simulink model "sl_braitenberg_1d"  (R2020b)
settings: Solver=VariableStepAuto  StartTime=0.0  StopTime=200  RelTol=1e-3  EnableMultiTasking=on
undefined symbols (not defined in the file or in its folder): SE2
libraries: roblocks x1, simulink x1
settings Model: Creator=corkep  LastModifiedBy=cr-ja
settings DataIOCC: LimitDataPoints=on  SaveFormat=Array  SaveOutput=off  SaveState=on  ReturnWorkspaceOutputs=off
settings OptimizationCC: LifeSpan=inf
settings DebuggingCC: AllowSymbolicDim=off  SFUnexpectedBacktrackingDiag=warning  SFNoUnconditionalDefaultTransitionDiag=warning  SFExecutionAtInitializationDiag=none  ArithmeticOperatorsInVariantConditions=warning
settings HardwareCC: ProdWordSize=32
settings ModelReferenceCC: PropagateSignalLabelsOutOfModel=off
settings SFSimCC: SimUseLocalCustomCode=off  CustomCodeUndefinedFunction=UseInterfaceOnly
settings RTWCC: RTWUseLocalCustomCode=off
settings CodeAppCC: StateflowObjectComments=on
settings GRTTargetCC: TargetLangStandard=C89/C90 (ANSI)
settings ConfigComp: CovMetricSettings=dw  CovSaveCumulativeToWorkspaceVar=on  CovSaveSingleToWorkspaceVar=on  CovExternalEMLEnable=off

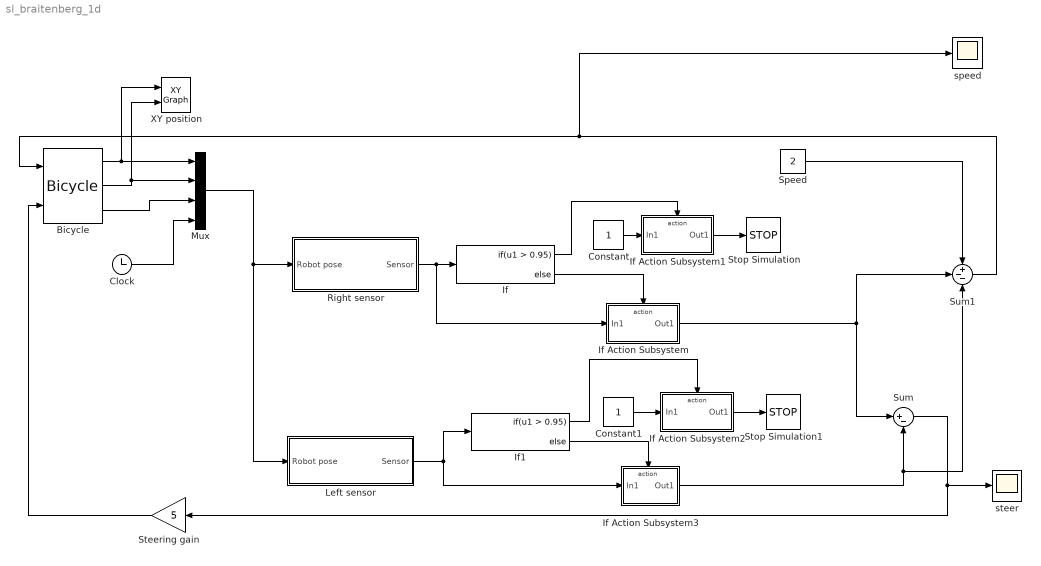
== system sl_braitenberg_1d ==
  Bicycle : roblocks/Vehicles/Bicycle  vlim=1  accel=1  alim=2  steer_rate=Inf  L=1  x0=[0, 0, 0]
  Clock : Clock
  Constant : Constant
  Constant1 : Constant
  If : If  IfExpression=u1 > 0.95
  If Action Subsystem : Subsystem  TreatAsAtomicUnit=on
  If Action Subsystem1 : Subsystem  TreatAsAtomicUnit=on
  If Action Subsystem2 : Subsystem  TreatAsAtomicUnit=on
  If Action Subsystem3 : Subsystem  TreatAsAtomicUnit=on
  If1 : If  IfExpression=u1 > 0.95
  Left sensor : Subsystem  mask{dx=0, dy=-2, sensorfunc=@sensorfield_1d}
      mask prompts: dx "Sensor position x"; dy "Sensor position y"; sensorfunc "Sensor function"
  Mux : Mux
  Right sensor : Subsystem  mask{dx=0, dy=2, sensorfunc=@sensorfield_1d}
      mask prompts: dx "Sensor position x"; dy "Sensor position y"; sensorfunc "Sensor function"
  Speed : Constant  Value=2
  Steering gain : Gain  Gain=5
  Stop Simulation : Stop
  Stop Simulation1 : Stop
  Sum : Sum  Inputs=|+-
  Sum1 : Sum  Inputs=+--
  XY position : simulink/Sinks/XY Graph  xmin=0  xmax=100  ymin=0  ymax=100  st=-1
  speed : Scope
  steer : Scope
  wires:
  Bicycle/1 -> XY position/1, Mux/1
  Bicycle/2 -> XY position/2, Mux/2
  Bicycle/3 -> Mux/3
  Mux/1 -> Left sensor/1(Robot pose), Right sensor/1(Robot pose)
  Sum/1 -> steer/1, Steering gain/1
  If Action Subsystem3/1(Out1) -> Sum/2, Sum1/3
  Sum1/1 -> Bicycle/1, speed/1
  Speed/1 -> Sum1/1
  Steering gain/1 -> Bicycle/2
  Clock/1 -> Mux/4
  If/1 -> If Action Subsystem1/Action
  If1/1 -> If Action Subsystem2/Action
  If Action Subsystem/1(Out1) -> Sum/1, Sum1/2
  If/2 -> If Action Subsystem/Action
  If Action Subsystem1/1(Out1) -> Stop Simulation/1
  Right sensor/1(Sensor) -> If Action Subsystem/1(In1), If/1
  If1/2 -> If Action Subsystem3/Action
  If Action Subsystem2/1(Out1) -> Stop Simulation1/1
  Left sensor/1(Sensor) -> If Action Subsystem3/1(In1), If1/1
  Constant/1 -> If Action Subsystem1/1(In1)
  Constant1/1 -> If Action Subsystem2/1(In1)

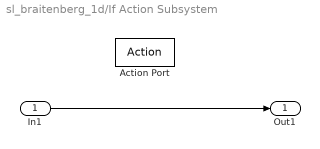
== system sl_braitenberg_1d/If Action Subsystem ==
  In1 : Inport
  Action Port : ActionPort  ActionPortLabel=else
  Out1 : Outport
  wires:
  In1/1 -> Out1/1

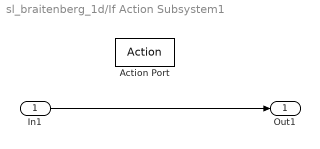
== system sl_braitenberg_1d/If Action Subsystem1 ==
  In1 : Inport
  Action Port : ActionPort  ActionPortLabel=if(u1 > 0.95)
  Out1 : Outport
  wires:
  In1/1 -> Out1/1

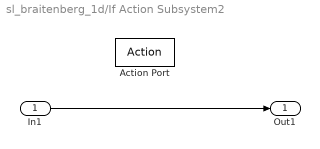
== system sl_braitenberg_1d/If Action Subsystem2 ==
  In1 : Inport
  Action Port : ActionPort  ActionPortLabel=if(u1 > 0.95)
  Out1 : Outport
  wires:
  In1/1 -> Out1/1

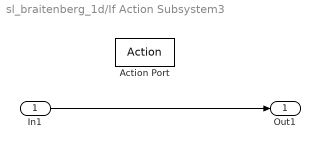
== system sl_braitenberg_1d/If Action Subsystem3 ==
  In1 : Inport
  Action Port : ActionPort  ActionPortLabel=else
  Out1 : Outport
  wires:
  In1/1 -> Out1/1

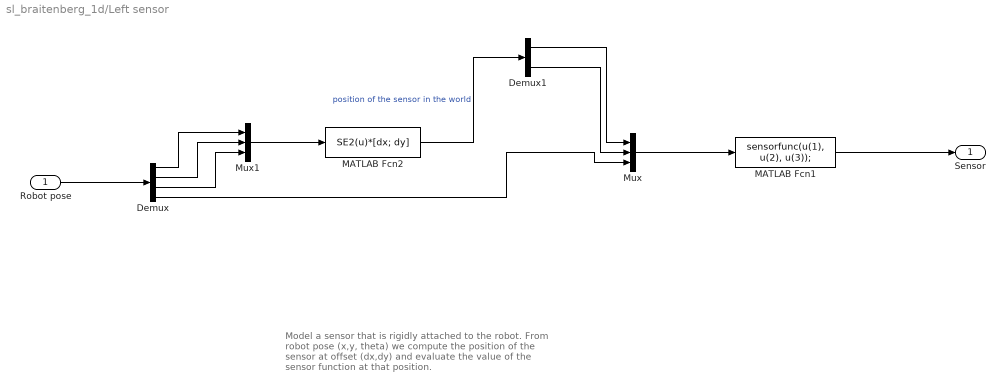
== system sl_braitenberg_1d/Left sensor ==
  note: Model a sensor that is rigidly attached to the robot.
      | From robot pose (x,y, theta) we compute the position of
      | the sensor at offset (dx,dy) and evaluate the value
      | of the sensor function at that position.
  Robot pose : Inport
  Demux : Demux
  Demux1 : Demux  Outputs=2
  MATLAB Fcn1 : MATLABFcn  MATLABFcn=sensorfunc(u(1), u(2), u(3));  OutputDimensions=1
  MATLAB Fcn2 : MATLABFcn  MATLABFcn=SE2(u)*[dx; dy]
  Mux : Mux  Inputs=3
  Mux1 : Mux  Inputs=3
  Sensor : Outport
  wires:
  MATLAB Fcn1/1 -> Sensor/1
  Demux/3 -> Mux1/3
  Demux1/1 -> Mux/1
  Demux/2 -> Mux1/2
  Demux/4 -> Mux/3
  Demux/1 -> Mux1/1
  Mux1/1 -> MATLAB Fcn2/1
  MATLAB Fcn2/1 -> Demux1/1  "position of the sensor in the world"
  Robot pose/1 -> Demux/1
  Mux/1 -> MATLAB Fcn1/1
  Demux1/2 -> Mux/2

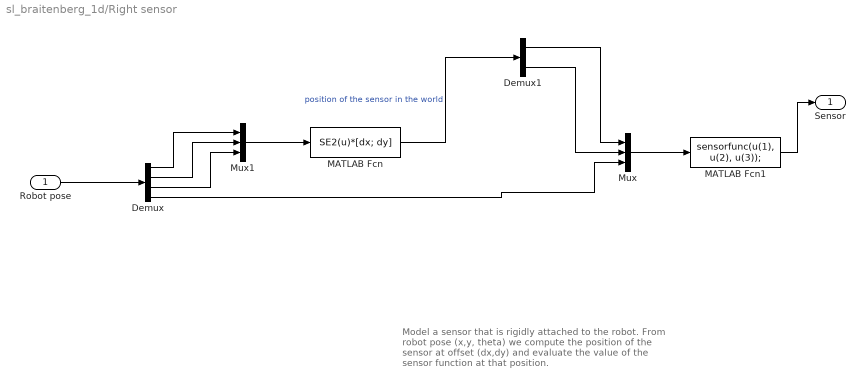
== system sl_braitenberg_1d/Right sensor ==
  note: Model a sensor that is rigidly attached to the robot.
      | From robot pose (x,y, theta) we compute the position of
      | the sensor at offset (dx,dy) and evaluate the value
      | of the sensor function at that position.
  Robot pose : Inport
  Demux : Demux
  Demux1 : Demux  Outputs=2
  MATLAB Fcn : MATLABFcn  MATLABFcn=SE2(u)*[dx; dy]
  MATLAB Fcn1 : MATLABFcn  MATLABFcn=sensorfunc(u(1), u(2), u(3));  OutputDimensions=1
  Mux : Mux  Inputs=3
  Mux1 : Mux  Inputs=3
  Sensor : Outport
  wires:
  MATLAB Fcn/1 -> Demux1/1  "position of the sensor in the world"
  MATLAB Fcn1/1 -> Sensor/1
  Robot pose/1 -> Demux/1
  Demux/1 -> Mux1/1
  Mux/1 -> MATLAB Fcn1/1
  Demux/3 -> Mux1/3
  Demux/2 -> Mux1/2
  Mux1/1 -> MATLAB Fcn/1
  Demux/4 -> Mux/3
  Demux1/2 -> Mux/2
  Demux1/1 -> Mux/1
